simulink model "retinasight_capacity_model"  (R2026a)
settings: Solver=ode45  StopTime=30
settings Model: Creator=mohan  LastModifiedBy=mohan

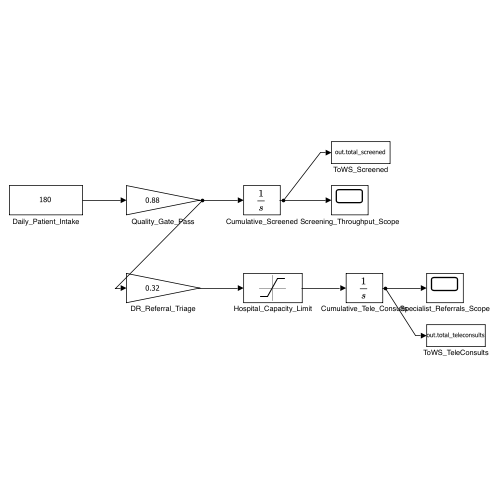
[thumbnail: Simulink's stored preview of the top-level diagram]
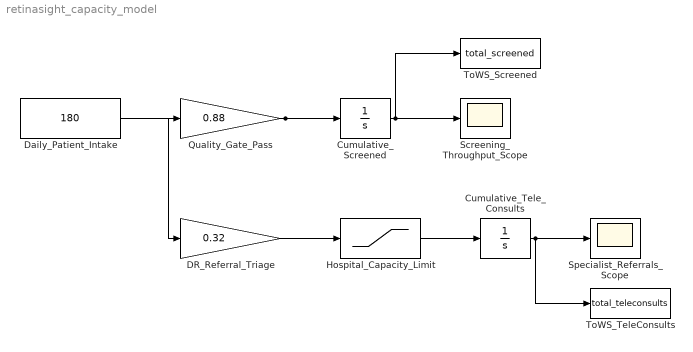
== system retinasight_capacity_model ==
  Cumulative_Screened : Integrator
  Cumulative_Tele_Consults : Integrator
  DR_Referral_Triage : Gain  Gain=0.32
  Daily_Patient_Intake : Constant  Value=180
  Hospital_Capacity_Limit : Saturate  UpperLimit=45  LowerLimit=0
  Quality_Gate_Pass : Gain  Gain=0.88
  Screening_Throughput_Scope : Scope
  Specialist_Referrals_Scope : Scope
  ToWS_Screened : ToWorkspace  VariableName=total_screened  SampleTime=-1
  ToWS_TeleConsults : ToWorkspace  VariableName=total_teleconsults  SampleTime=-1
  wires:
  Daily_Patient_Intake/1 -> Quality_Gate_Pass/1
  Quality_Gate_Pass/1 -> Cumulative_Screened/1, DR_Referral_Triage/1
  Cumulative_Screened/1 -> Screening_Throughput_Scope/1, ToWS_Screened/1
  DR_Referral_Triage/1 -> Hospital_Capacity_Limit/1
  Hospital_Capacity_Limit/1 -> Cumulative_Tele_Consults/1
  Cumulative_Tele_Consults/1 -> Specialist_Referrals_Scope/1, ToWS_TeleConsults/1
